simulink model "anglefiltering"  (R2024b)
settings: Solver=FixedStepAuto  StartTime=0.0  StopTime=simDuration  FixedStep=0.01  RelTol=1e-3
undefined symbols (not defined in the file or in its folder): K
libraries: simulink x2, arduinosensorlib x2, dspswit3 x1, dspfdesign x1
settings Model: Creator=ARIES  LastModifiedBy=zglin

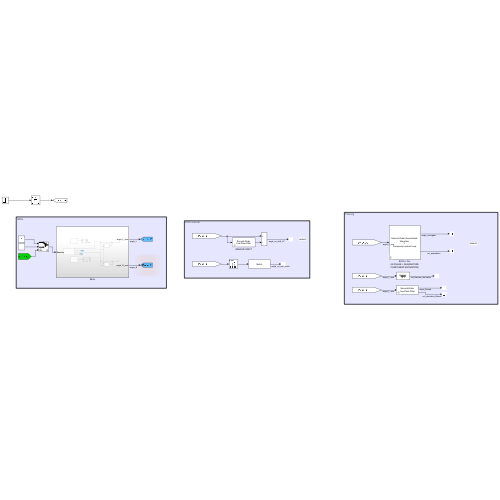
[thumbnail: Simulink's stored preview of the top-level diagram]
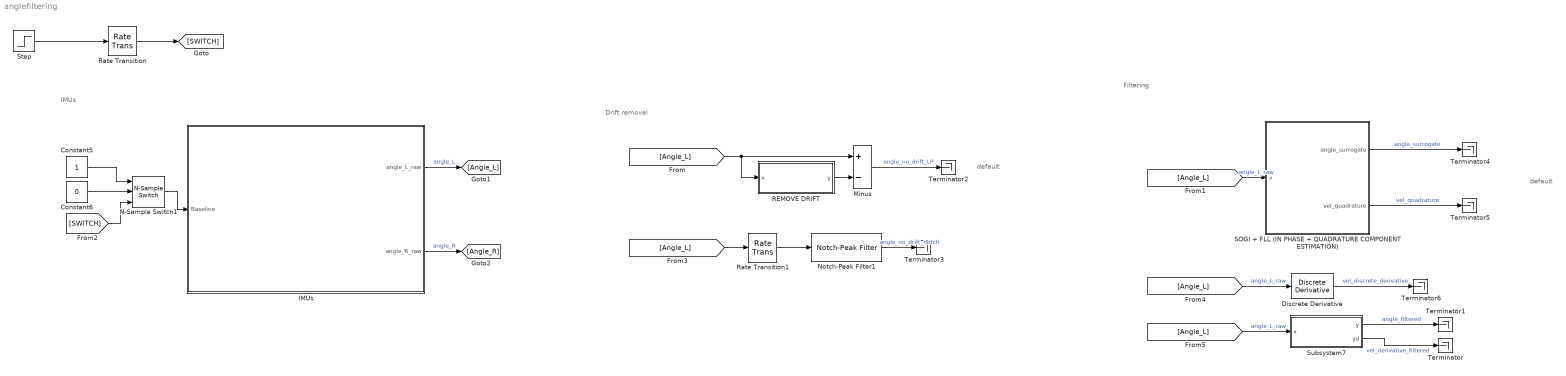
== system anglefiltering ==
  note: default
  note: default
  note: Drift removal
  note: IMUs
  note: Filtering
  Constant5 : Constant
  Constant6 : Constant  Value=0
  Discrete Derivative : simulink/Discrete/Discrete Derivative  gainval=1.0  ICPrevScaledInput=0.0  OutMin=[]  OutMax=[]  OutDataType=fixdt(1, 16)  OutScaling=2^-10  DoSatur=off
  IMUs : Subsystem
  Minus : Sum  Inputs=+-
  N-Sample Switch1 : dspswit3/N-Sample Switch  N=10  reset=on  TriggerType=Rising edge  Ts=0.01
  Notch-Peak Filter1 : dspfdesign/Notch-Peak Filter  Specification=Bandwidth and center frequency  BandwidthPort=off  Bandwidth=0.1  QualityFactorPort=off  QualityFactor=5  CenterFrequencyPort=off  CenterFrequency=0  BandwidthCoefficientPort=off  BandwidthCoefficient=0.72654  CenterFrequencyCoefficientPort=off  CenterFrequencyCoefficient=0  Output=Notch  SampleRateMode=Specify on dialog  SampleRate=100  SimulateUsing=Interpreted execution
  REMOVE DRIFT : Subsystem  mask{wn=1.25, zt=1, x0=0}
      mask prompts: wn "Cut-off frequency (rad/s)"; zt "Damping ratio"; x0 "Initial Condition"
      mask Display: disp('Second-Order\nLow-Pass Filter');
  Rate Transition : RateTransition  OutPortSampleTime=0.01
  Rate Transition1 : RateTransition  OutPortSampleTime=0.01
  SOGI + FLL (IN PHASE + QUADRATURE COMPONENT ESTIMATION) : Subsystem  mask{Tsamp=0.01, fmin=0.2, fmax=4.0, ksogi=1, kfll=1.0, Elo=1e-4, Ehi=1e-2}
      mask prompts: Tsamp "Sampling time (s)"; fmin "Minimum movement frequency (Hz)"; fmax "Maximum movement frequency (Hz)"; ksogi "SOGI amplitude adaptation gain"; kfll "FLL frequency adaptation gain"; Elo "Low energy threshold"; Ehi "High energy threshold"
      mask Display: disp('Second-Order Generalized \nIntegrator \n+ \nFrequency-Locked Loop');
  Step : Step  SampleTime=0
  Subsystem7 : Subsystem  mask{wn=100, zt=1, x0=0}
      mask prompts: wn "Cut-off frequency (rad/s)"; zt "Damping ratio"; x0 "Initial Condition"
      mask Display: disp('Second-Order\nLow-Pass Filter');
  Terminator{,1..6} (7 alike) : Terminator
  wires:
  Constant5/1 -> N-Sample Switch1/1
  N-Sample Switch1/1 -> IMUs/1(Baseline)
  Constant6/1 -> N-Sample Switch1/2
  IMUs/2(angle_R_raw) -> [Angle_R]  "angle_R"
  IMUs/1(angle_L_raw) -> [Angle_L]  "angle_L"
  [SWITCH] -> N-Sample Switch1/3
  Subsystem7/1(y) -> Terminator1/1  "angle_filtered"
  SOGI + FLL (IN PHASE + QUADRATURE COMPONENT ESTIMATION)/2(vel_quadrature) -> Terminator5/1  "vel_quadrature"
  SOGI + FLL (IN PHASE + QUADRATURE COMPONENT ESTIMATION)/1(angle_surrogate) -> Terminator4/1  "angle_surrogate"
  [Angle_L] -> SOGI + FLL (IN PHASE + QUADRATURE COMPONENT ESTIMATION)/1(x)  "angle_L_raw"
  [Angle_L] -> Minus/1, REMOVE DRIFT/1(x)
  REMOVE DRIFT/1(y) -> Minus/2
  Subsystem7/2(yd) -> Terminator/1  "vel_derivative_filtered"
  Minus/1 -> Terminator2/1  "angle_no_drift_LP"
  [Angle_L] -> Rate Transition1/1
  Notch-Peak Filter1/1 -> Terminator3/1  "angle_no_drift_notch"
  Discrete Derivative/1 -> Terminator6/1  "vel_discrete_derivative"
  [Angle_L] -> Subsystem7/1(x)  "angle_L_raw"
  [Angle_L] -> Discrete Derivative/1  "angle_L_raw"
  Step/1 -> Rate Transition/1
  Rate Transition/1 -> [SWITCH]
  Rate Transition1/1 -> Notch-Peak Filter1/1

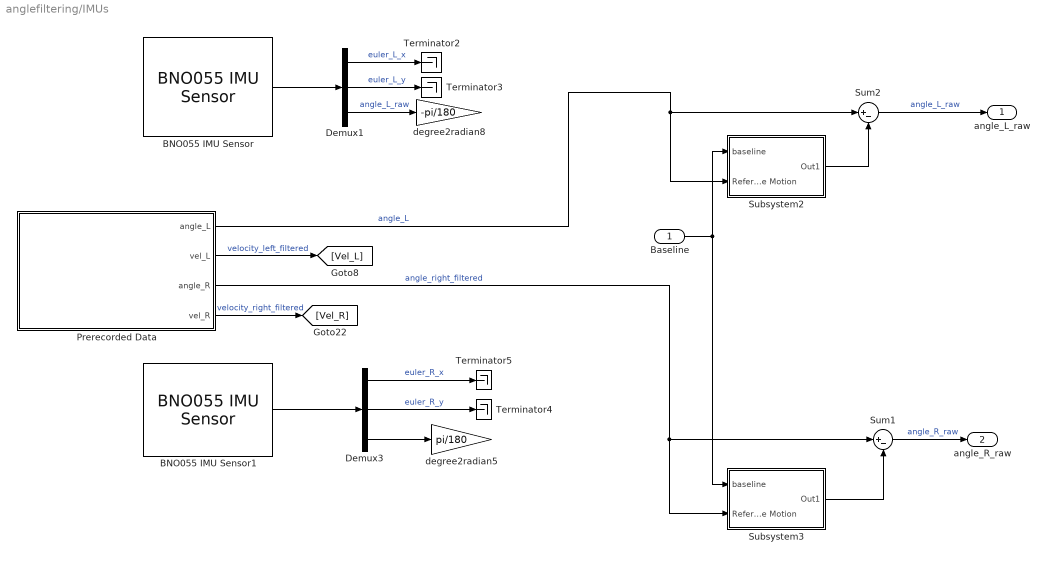
== system anglefiltering/IMUs ==
  Baseline : Inport
  BNO055 IMU Sensor : arduinosensorlib/BNO055 IMU Sensor  I2CModule=0  SlaveAddress=0x28  OperationMode=Fusion  Accel=off  AngularRate=off  MagField=off  EulerAngles=on  Quat=off  LinearAccel=off  GravityVector=off  Status=off  Timestamp=off  AccelRange=4G  AccelBW=62.5 Hz  GyroRange=2000 dps  GyroBW=32 Hz  MagODR=10 Hz  spf=1  SampleTime=-1  blockPlatform=ARDUINO  QueueSizeFactor=1
      settings: SourceProductName=Sensors
  BNO055 IMU Sensor1 : arduinosensorlib/BNO055 IMU Sensor  I2CModule=0  SlaveAddress=0x29  OperationMode=Fusion  Accel=off  AngularRate=off  MagField=off  EulerAngles=on  Quat=off  LinearAccel=off  GravityVector=off  Status=off  Timestamp=off  AccelRange=4G  AccelBW=62.5 Hz  GyroRange=2000 dps  GyroBW=32 Hz  MagODR=10 Hz  spf=1  SampleTime=-1  blockPlatform=ARDUINO  QueueSizeFactor=1
      settings: SourceProductName=Sensors
  Demux1 : Demux  Outputs=3
  Demux3 : Demux  Outputs=3
  Prerecorded Data : Subsystem
  Subsystem2 : Subsystem
  Subsystem3 : Subsystem
  Sum1 : Sum  Inputs=|+-
  Sum2 : Sum  Inputs=|+-
  Terminator{2..5} (4 alike) : Terminator
  degree2radian5 : Gain  Gain=pi/180
  degree2radian8 : Gain  Gain=-pi/180
  angle_L_raw : Outport
  angle_R_raw : Outport  Port=2
  wires:
  BNO055 IMU Sensor/1 -> Demux1/1
  BNO055 IMU Sensor1/1 -> Demux3/1
  Demux1/1 -> Terminator2/1  "euler_L_x"
  Demux1/3 -> degree2radian8/1  "angle_L_raw"
  Demux1/2 -> Terminator3/1  "euler_L_y"
  Demux3/1 -> Terminator5/1  "euler_R_x"
  Demux3/2 -> Terminator4/1  "euler_R_y"
  Demux3/3 -> degree2radian5/1
  Baseline/1 -> Subsystem2/1(baseline), Subsystem3/1(baseline)
  Subsystem2/1(Out1) -> Sum2/2
  Subsystem3/1(Out1) -> Sum1/2
  Prerecorded Data/1(angle_L) -> Subsystem2/2(Reference Motion), Sum2/1  "angle_L"
  Sum2/1 -> angle_L_raw/1  "angle_L_raw"
  Sum1/1 -> angle_R_raw/1  "angle_R_raw"
  Prerecorded Data/4(vel_R) -> [Vel_R]  "velocity_right_filtered"
  Prerecorded Data/3(angle_R) -> Subsystem3/2(Reference Motion), Sum1/1  "angle_right_filtered"
  Prerecorded Data/2(vel_L) -> [Vel_L]  "velocity_left_filtered"

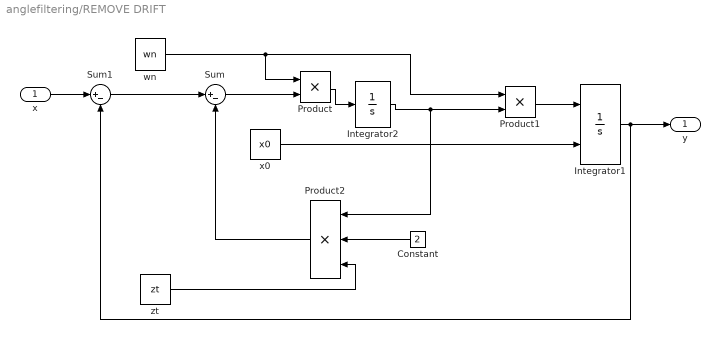
== system anglefiltering/REMOVE DRIFT ==
  x : Inport
  Constant : Constant  Value=2
  Integrator1 : Integrator  InitialConditionSource=external
  Integrator2 : Integrator
  Product : Product  RndMeth=Zero
  Product1 : Product  RndMeth=Zero
  Product2 : Product  Inputs=3  RndMeth=Zero
  Sum : Sum  Inputs=|+-
  Sum1 : Sum  Inputs=|+-
  wn : Constant  Value=wn
  x0 : Constant  Value=x0
  zt : Constant  Value=zt
  y : Outport  VectorParamsAs1DForOutWhenUnconnected=off
  wires:
  Sum/1 -> Product/2
  wn/1 -> Product/1, Product1/1
  Sum1/1 -> Sum/1
  x0/1 -> Integrator1/2
  Integrator2/1 -> Product1/2, Product2/1
  Product/1 -> Integrator2/1
  x/1 -> Sum1/1
  Product1/1 -> Integrator1/1
  Integrator1/1 -> Sum1/2, y/1
  Product2/1 -> Sum/2
  zt/1 -> Product2/3
  Constant/1 -> Product2/2

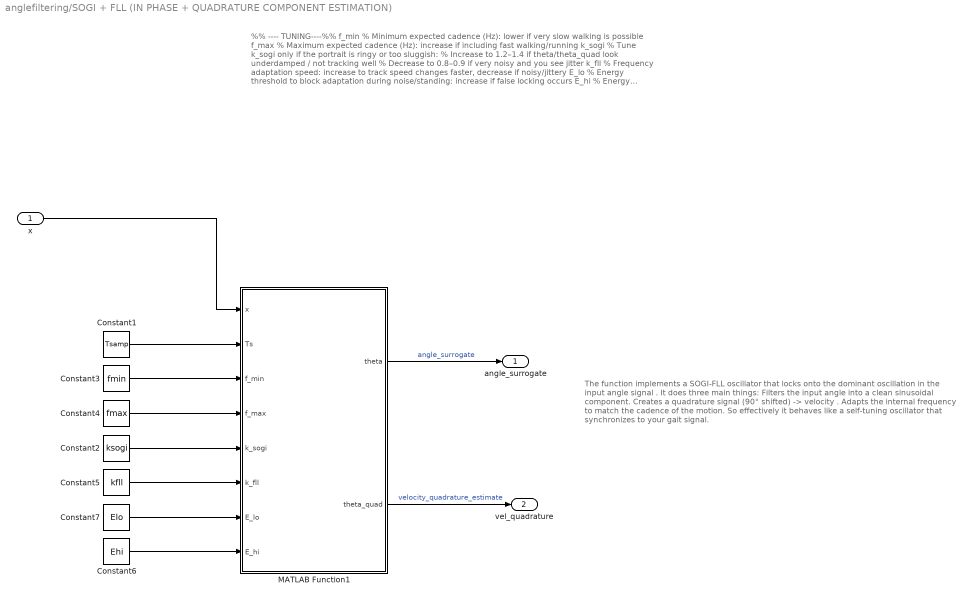
== system anglefiltering/SOGI + FLL (IN PHASE + QUADRATURE COMPONENT ESTIMATION) ==
  note: The function implements a SOGI-FLL oscillator that locks onto the dominant oscillation in the input angle signal . It does three main things:
      | Filters the input angle into a clean sinusoidal component.
      | Creates a quadrature signal (90° shifted) -> velocity .
      | Adapts the internal frequency to match the cadence of the motion.
      | So effectively it behaves like a self-tuning oscillator that synchronizes to your gait signal.
  note: %% ---- TUNING----%%
      |
      | f_min % Minimum expected cadence (Hz): lower if very slow walking is possible
      | f_max % Maximum expected cadence (Hz): increase if including fast walking/running
      |
      | k_sogi % Tune k_sogi only if the portrait is ringy or too sluggish:
      | % Increase to 1.2–1.4 if theta/theta_quad look underdamped / not tracking well
      | % Decrease to 0.8–0.9 if very noisy and you see jitter
      |
      | k_fll % Frequency adaptation speed: increase to track speed changes faster, decrease if noisy/jittery
      |
      | E_lo % Energy threshold to block adaptation during noise/standing: increase if false locking occurs
      | E_hi % Energy threshold for full adaptation: decrease if it never locks during slow gait
      |
      | OTHER PARAMETERS TO BE TUNED INSIDE THE MATLAB FUNCTION (for walking/running there should not be the need)
  x : Inport
  Constant1 : Constant  Value=Tsamp
  Constant2 : Constant  Value=ksogi
  Constant3 : Constant  Value=fmin
  Constant4 : Constant  Value=fmax
  Constant5 : Constant  Value=kfll
  Constant6 : Constant  Value=Ehi
  Constant7 : Constant  Value=Elo
  MATLAB Function1 : MATLAB Function  TreatAsAtomicUnit=on
  angle_surrogate : Outport
  vel_quadrature : Outport  Port=2
  wires:
  x/1 -> MATLAB Function1/1(x)
  Constant3/1 -> MATLAB Function1/3(f_min)
  Constant4/1 -> MATLAB Function1/4(f_max)
  Constant5/1 -> MATLAB Function1/6(k_fll)
  Constant6/1 -> MATLAB Function1/8(E_hi)
  Constant1/1 -> MATLAB Function1/2(Ts)
  Constant7/1 -> MATLAB Function1/7(E_lo)
  Constant2/1 -> MATLAB Function1/5(k_sogi)
  MATLAB Function1/1(theta) -> angle_surrogate/1  "angle_surrogate"
  MATLAB Function1/2(theta_quad) -> vel_quadrature/1  "velocity_quadrature_estimate"

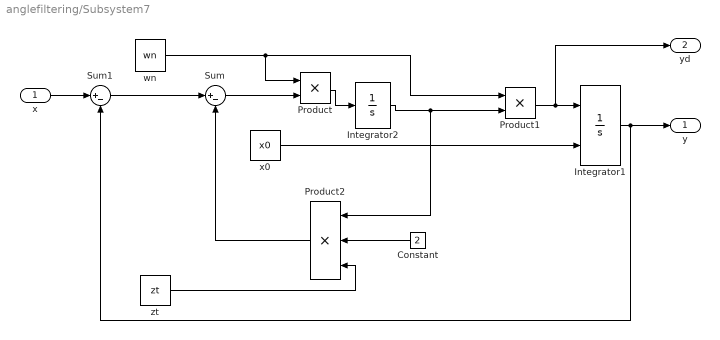
== system anglefiltering/Subsystem7 ==
  x : Inport
  Constant : Constant  Value=2
  Integrator1 : Integrator  InitialConditionSource=external
  Integrator2 : Integrator
  Product : Product  RndMeth=Zero
  Product1 : Product  RndMeth=Zero
  Product2 : Product  Inputs=3  RndMeth=Zero
  Sum : Sum  Inputs=|+-
  Sum1 : Sum  Inputs=|+-
  wn : Constant  Value=wn
  x0 : Constant  Value=x0
  zt : Constant  Value=zt
  y : Outport  VectorParamsAs1DForOutWhenUnconnected=off
  yd : Outport  Port=2  VectorParamsAs1DForOutWhenUnconnected=off
  wires:
  Sum/1 -> Product/2
  wn/1 -> Product/1, Product1/1
  Sum1/1 -> Sum/1
  x0/1 -> Integrator1/2
  Integrator2/1 -> Product1/2, Product2/1
  Product/1 -> Integrator2/1
  x/1 -> Sum1/1
  Product1/1 -> Integrator1/1, yd/1
  Integrator1/1 -> Sum1/2, y/1
  Product2/1 -> Sum/2
  zt/1 -> Product2/3
  Constant/1 -> Product2/2

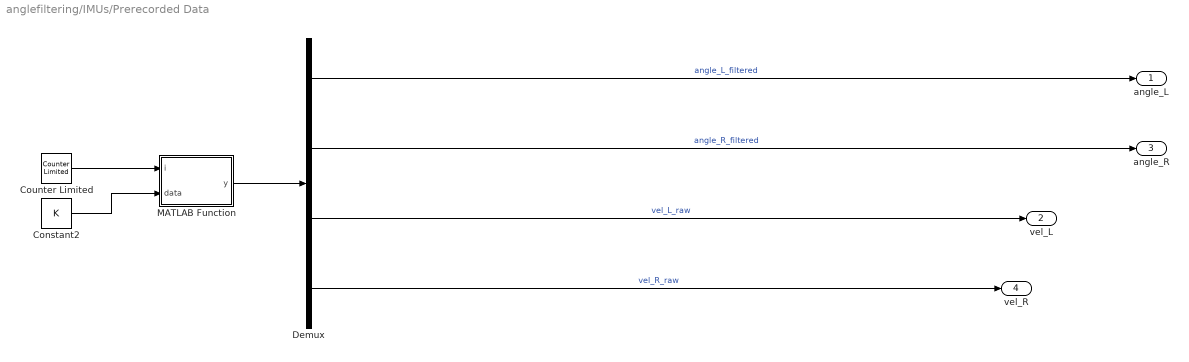
== system anglefiltering/IMUs/Prerecorded Data ==
  Constant2 : Constant  Value=K
  Counter Limited : simulink/Sources/Counter Limited  uplimit=size(K,1)  tsamp=0.01
  Demux : Demux
  MATLAB Function : MATLAB Function  TreatAsAtomicUnit=on
  angle_L : Outport
  vel_L : Outport  Port=2
  angle_R : Outport  Port=3
  vel_R : Outport  Port=4
  wires:
  MATLAB Function/1(y) -> Demux/1
  Counter Limited/1 -> MATLAB Function/1(i)
  Constant2/1 -> MATLAB Function/2(data)
  Demux/2 -> angle_R/1  "angle_R_filtered"
  Demux/1 -> angle_L/1  "angle_L_filtered"
  Demux/3 -> vel_L/1  "vel_L_raw"
  Demux/4 -> vel_R/1  "vel_R_raw"

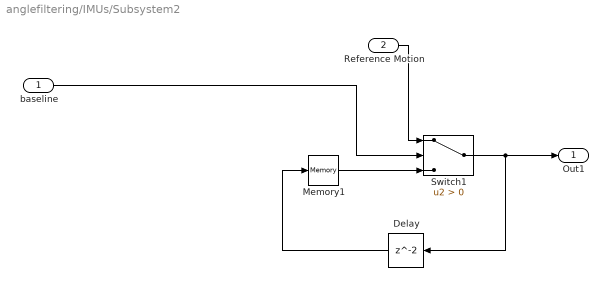
== system anglefiltering/IMUs/Subsystem2 ==
  baseline : Inport
  Reference Motion : Inport  Port=2
  Delay : Delay
  Memory1 : Memory
  Switch1 : Switch  Criteria=u2 > Threshold  SaturateOnIntegerOverflow=off  InputSameDT=off
  Out1 : Outport
  wires:
  Switch1/1 -> Delay/1, Out1/1
  Memory1/1 -> Switch1/3
  baseline/1 -> Switch1/2
  Reference Motion/1 -> Switch1/1
  Delay/1 -> Memory1/1

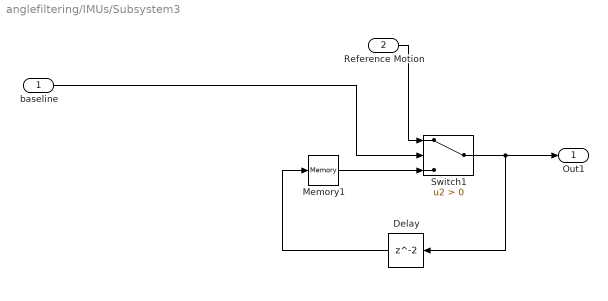
== system anglefiltering/IMUs/Subsystem3 ==
  baseline : Inport
  Reference Motion : Inport  Port=2
  Delay : Delay
  Memory1 : Memory
  Switch1 : Switch  Criteria=u2 > Threshold  SaturateOnIntegerOverflow=off  InputSameDT=off
  Out1 : Outport
  wires:
  Switch1/1 -> Delay/1, Out1/1
  Memory1/1 -> Switch1/3
  baseline/1 -> Switch1/2
  Reference Motion/1 -> Switch1/1
  Delay/1 -> Memory1/1

== matlab function anglefiltering/SOGI + FLL (IN PHASE + QUADRATURE COMPONENT ESTIMATION)/MATLAB Function1 ==
  settings: updateMethod=DISCRETE
  data: x input; Ts input; f_min input; f_max input; theta output; k_sogi input; theta_quad output; k_fll input; E_lo input; E_hi input
function [theta, theta_quad] = SOGI_FLL( ...
    x, Ts, ...
    f_min, f_max, ...     % cadence bounds (walking/running range)
    k_sogi, k_fll, ...            % FLL adaptation speed (sensor/noise dependent)
    E_lo, E_hi)           % lock thresholds (amplitude/noise dependent)


% SOGI-FLL:
%   SOGI = Second-Order Generalized Integrator (generates in-phase + quadrature)
%   FLL  = Frequency-Locked Loop (adapts internal frequency to cadence changes)
%
% INPUTS:
%   x       : drift-removed joint angle [rad] (recommended: x = theta_raw - slowLPF(theta_raw))
%   walking : boolean gate (true when moving; false when standing)
%   Ts      : sample time [s]
%
%   f_min,f_max : [Hz] plausible cadence bounds (include running if needed)
%   k_fll       : FLL adaptation gain (higher=faster, more sensitive to noise)
%   E_lo,E_hi   : energy thresholds for confidence/lock (depends on amplitude & noise)
%
% OUTPUTS:
%   theta       : in-phase filtered signal
%   theta_quad  : quadrature signal

%% -------- Fixed “rarely changed” parameters (keep inside) --------

walking = 1.0; %walking detected

fc_f_smooth = 0.30;
% Tune only if internal frequency becomes jittery or too laggy:
%   - decrease to 0.2 for smoother (more lag)
%   - increase to 0.5 for faster (more jitter)

fc_lock = 0.50;
% Tune only if lock flickers or reacts too slowly:
%   - decrease (0.3) to reduce flicker
%   - increase (0.8–1.0) for faster start/stop response

f_init = 1.4;              % [Hz] initial guess (walking/running general default)
% Tune only if you want faster lock at startup:
%   - set near typical cadence in your trials (walk ~1–2 Hz, run ~2–3 Hz)

decay_notwalking = 0.999;   % state decay when standing
% Tune only if oscillator rings too long after stopping:
%   - faster decay: 0.995
%   - slower decay: 0.9995

epsSmall = 1e-9;            % numerical safety
% Increase only if you see NaN/Inf in extreme low-motion segments (e.g., 1e-8)

%% -------------------- Persistent states --------------------
persistent va vb w_est f_state lock_state
if isempty(va)
    va = 0; vb = 0;
    w_est = 2*pi*f_init;
    f_state = f_init;
    lock_state = 0;
end

%% -------------------- Precompute smoothing coefficients --------------------
aF    = exp(-2*pi*fc_f_smooth*Ts);
aLock = exp(-2*pi*fc_lock*Ts);

%% -------------------- Frequency bounds in rad/s --------------------
w_min = 2*pi*f_min;
w_max = 2*pi*f_max;

w0 = clamp(w_est, w_min, w_max);

%% ==================== SOGI ====================
if walking
    e = x - va;

    va = va + Ts*( w0*vb + k_sogi*w0*e );
    vb = vb + Ts*( -w0*va );
else
    va = decay_notwalking*va;
    vb = decay_notwalking*vb;
    e  = 0;
end

theta = va;
theta_quad = vb;

%% ==================== Lock/confidence ====================
E = theta*theta + theta_quad*theta_quad;
lock_state = aLock*lock_state + (1-aLock)*E;

lock = clamp((lock_state - E_lo)/(E_hi - E_lo + epsSmall), 0, 1);

%% ==================== FLL ====================
if walking
    mu = (e * theta_quad) / (E + epsSmall);

    w_est = w0 + Ts * (k_fll * w0 * mu) * lock;
    w_est = clamp(w_est, w_min, w_max);

    f_raw = w_est/(2*pi);
    f_state = aF*f_state + (1-aF)*f_raw;

    w_est = 2*pi*clamp(f_state, f_min, f_max);
else
    f_state = 0.995*f_state + 0.005*f_init;
    w_est   = 2*pi*f_state;
end

end

function y = clamp(x, lo, hi)
y = min(max(x, lo), hi);
end

== matlab function anglefiltering/IMUs/Prerecorded Data/MATLAB Function ==
  data: i input; y output; data input
function y = imuPlayback(i, data)
%#codegen
% imuData must be defined as a Simulink.Parameter in the base workspace.
% Example: imuData = Simulink.Parameter(yourIMUArray);
% y will be a 1x4 row vector
if i+1 <= size(data,1)
    y = data(i+1,:);      % pick row i
else
    y = data(end,:);    % after end, hold last value
end
end
